simulink model "tricycle_v2"  (R2016a)
settings: Solver=FixedStepAuto  StartTime=0.0  StopTime=50  FixedStep=0.1  RelTol=1e-3
values from neighbouring files (symbols this model uses):
  gamma_max = pi/4    (= 0.785398163397)    [parameter.m]
  v_max = 1.5 + 0.03*g    (= 1.68)    [parameter.m]
libraries: simulink x5
settings Model: Creator=Nam Bui Duy  LastModifiedBy=Nam Bui Duy

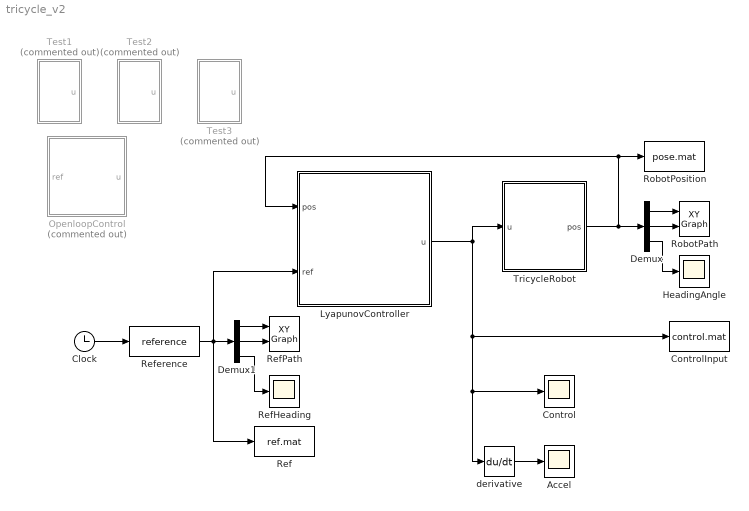
== system tricycle_v2 ==
  Accel : Scope
  Clock : Clock
  Control : Scope
  ControlInput : ToFile  Filename=control.mat  SaveFormat=Timeseries
  Demux : Demux  Outputs=3
  Demux1 : Demux  Outputs=3
  HeadingAngle : Scope
  LyapunovController : Subsystem
  OpenloopControl : Subsystem  Commented=on
  Ref : ToFile  Filename=ref.mat  SaveFormat=Timeseries
  RefHeading : Scope
  RefPath : simulink/Sinks/XY Graph  xmin=-21  xmax=5  ymin=-5  ymax=5  st=-1
  Reference : MATLABFcn  MATLABFcn=reference  OutputDimensions=3
  RobotPath : simulink/Sinks/XY Graph  xmin=-21  xmax=5  ymin=-5  ymax=5  st=-1
  RobotPosition : ToFile  Filename=pose.mat  SaveFormat=Timeseries
  Test1 : Subsystem  Commented=on
  Test2 : Subsystem  Commented=on
  Test3 : Subsystem  Commented=on
  TricycleRobot : Subsystem
  derivative : Derivative
  wires:
  TricycleRobot/1(pos) -> RobotPosition/1, LyapunovController/1(pos), Demux/1
  Demux/1 -> RobotPath/1
  Demux/2 -> RobotPath/2
  Demux/3 -> HeadingAngle/1
  Clock/1 -> Reference/1
  Reference/1 -> LyapunovController/2(ref), Demux1/1, Ref/1
  Demux1/1 -> RefPath/1
  Demux1/2 -> RefPath/2
  derivative/1 -> Accel/1
  Demux1/3 -> RefHeading/1
  LyapunovController/1(u) -> TricycleRobot/1(u), derivative/1, Control/1, ControlInput/1

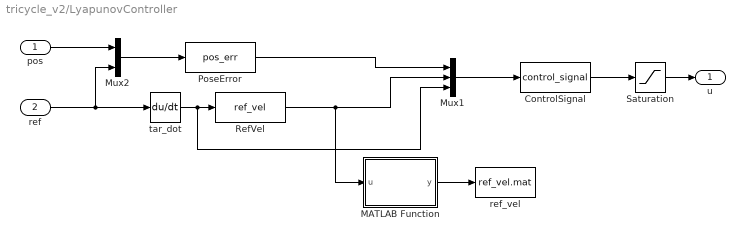
== system tricycle_v2/LyapunovController ==
  pos : Inport
  ref : Inport  Port=2
  ControlSignal : MATLABFcn  MATLABFcn=control_signal  OutputDimensions=2
  MATLAB Function : MATLAB Function  TreatAsAtomicUnit=on
  Mux1 : Mux  Inputs=3
  Mux2 : Mux  Inputs=2
  PoseError : MATLABFcn  MATLABFcn=pos_err  OutputDimensions=3
  RefVel : MATLABFcn  MATLABFcn=ref_vel  OutputDimensions=2
  Saturation : Saturate  UpperLimit=[v_max; gamma_max]  LowerLimit=-[v_max; gamma_max]
  ref_vel : ToFile  Filename=ref_vel.mat  SaveFormat=Timeseries
  tar_dot : Derivative
  u : Outport
  wires:
  Mux1/1 -> ControlSignal/1
  ref/1 -> Mux2/2, tar_dot/1
  pos/1 -> Mux2/1
  RefVel/1 -> MATLAB Function/1(u), Mux1/2
  ControlSignal/1 -> Saturation/1
  PoseError/1 -> Mux1/1
  Mux2/1 -> PoseError/1
  tar_dot/1 -> Mux1/3, RefVel/1
  Saturation/1 -> u/1
  MATLAB Function/1(y) -> ref_vel/1

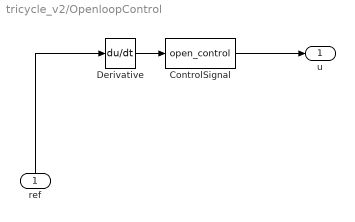
== system tricycle_v2/OpenloopControl ==
  ref : Inport
  ControlSignal : MATLABFcn  MATLABFcn=open_control  OutputDimensions=2
  Derivative : Derivative
  u : Outport
  wires:
  ControlSignal/1 -> u/1
  ref/1 -> Derivative/1
  Derivative/1 -> ControlSignal/1

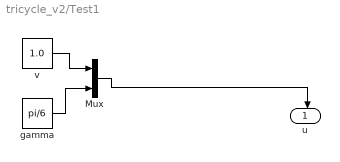
== system tricycle_v2/Test1 ==
  Mux : Mux  Inputs=2
  gamma : Constant  Value=pi/6
  v : Constant  Value=1.0
  u : Outport
  wires:
  Mux/1 -> u/1
  gamma/1 -> Mux/2
  v/1 -> Mux/1

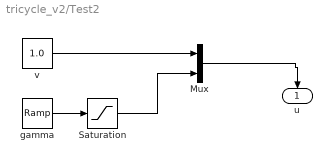
== system tricycle_v2/Test2 ==
  Mux : Mux  Inputs=2
  Saturation : Saturate  UpperLimit=gamma_max  LowerLimit=-gamma_max
  gamma : simulink/Sources/Ramp  slope=0.5  start=0  X0=0
  v : Constant  Value=1.0
  u : Outport
  wires:
  Mux/1 -> u/1
  v/1 -> Mux/1
  gamma/1 -> Saturation/1
  Saturation/1 -> Mux/2

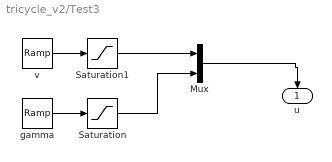
== system tricycle_v2/Test3 ==
  Mux : Mux  Inputs=2
  Saturation : Saturate  UpperLimit=gamma_max  LowerLimit=-gamma_max
  Saturation1 : Saturate  UpperLimit=v_max  LowerLimit=-v_max
  gamma : simulink/Sources/Ramp  slope=0.5  start=0  X0=0
  v : simulink/Sources/Ramp  slope=0.2  start=0  X0=0
  u : Outport
  wires:
  Mux/1 -> u/1
  Saturation1/1 -> Mux/1
  gamma/1 -> Saturation/1
  Saturation/1 -> Mux/2
  v/1 -> Saturation1/1

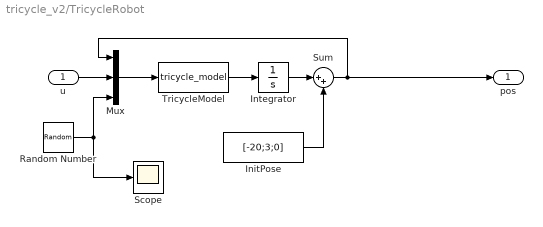
== system tricycle_v2/TricycleRobot ==
  u : Inport
  InitPose : Constant  Value=[-20;3;0]
  Integrator : Integrator
  Mux : Mux  Inputs=3
  Random Number : RandomNumber  Variance=0  SampleTime=0.1
  Scope : Scope
  Sum : Sum  Inputs=|++
  TricycleModel : MATLABFcn  MATLABFcn=tricycle_model  OutputDimensions=3
  pos : Outport
  wires:
  Mux/1 -> TricycleModel/1
  u/1 -> Mux/2
  TricycleModel/1 -> Integrator/1
  Integrator/1 -> Sum/1
  InitPose/1 -> Sum/2
  Sum/1 -> pos/1, Mux/1
  Random Number/1 -> Scope/1, Mux/3

== matlab function tricycle_v2/LyapunovController/MATLAB Function ==
  data: u input; y output
function y = fcn(u)
%#codegen
d = 1.8166;
v = u(1);
gamma = atan2(u(2)*d, v);
y = [v; gamma];
